simulink model "c221106_FCEV_SLMP_SQP"  (R2022b)
settings: Solver=FixedStepAuto  StartTime=0.0  StopTime=DrvCycLen  FixedStep=1  RelTol=1e-3
values from neighbouring files (symbols this model uses):
  AccThrshd = 1    [Config_c221112.m]    (also in Config_c221127.m; Config_c221218.m; Config_c230117.m; Config_c230321.m)
  AlphaRampFactor = 8    [Config_c221112.m]    (also in Config_c221127.m; Config_c221218.m; Config_c230117.m; Config_c230321.m)
  Bat_eff_chg_average = 0.969    [FCEV_original_data.mat]
  Bat_eff_dis_average = 0.9632    [FCEV_original_data.mat]
  Bat_end_of_life_percent = 20    [FCEV_original_data.mat]
  Bat_I_chg_max = -120    [FCEV_original_data.mat]
  Bat_I_dis_max = 200    [FCEV_original_data.mat]
  Bat_nom_Ic = 2.5    [FCEV_original_data.mat]
  Bat_nom_SOC = 0.35    [FCEV_original_data.mat]
  Bat_nom_temp_oC = 25    [FCEV_original_data.mat]
  Bat_num_pa = 9    [FCEV_original_data.mat]
  Bat_num_se = 97    [FCEV_original_data.mat]
  Bat_ori_C1_chg_F = [397.526659684 455.660832136 435.08783522 460.845064365 457.605812374 417.289828504 416.373906992 359.741413056 321.561704819 1109.14132554 1165.67733205 1135.97600211 ... (72 elements, 9x8)]    [FCEV_original_data.mat]
  Bat_ori_C1_dis_F = [187.121968588 287.083505726 346.448009002 395.529439835 387.517274826 389.973134196 432.856765051 486.92921923 512.158935268 425.990733989 614.68708868 771.472592368 ... (72 elements, 9x8)]    [FCEV_original_data.mat]
  Bat_ori_C2_chg_F = [8748.48589695 7773.35875681 9404.86567646 8934.73981058 8290.58671366 7592.78422269 7759.44623103 7396.59043829 6151.35152293 16187.7227039 11721.8480541 13157.8579836 ... (72 elements, 9x8)]    [FCEV_original_data.mat]
  Bat_ori_C2_dis_F = [2939.81325553 4590.73311898 5504.93546413 5887.5077374 6534.37836712 7765.46899768 10584.7751706 10372.0508438 9238.72693885 5207.86390693 7911.43744944 8879.62137571 ... (72 elements, 9x8)]    [FCEV_original_data.mat]
  Bat_ori_cap_max_Ah = 20.7    [Config_c221218.m]    (also in Config_c230117.m; Config_c230321.m; FCEV_original_data.mat)
  Bat_ori_dUdt4 = [-0.303773584906 -0.249056603774 -0.115094339623 -0.0396226415094 0.0396226415094 0.0641509433962 0.107547169811 0.111320754717 0.0415094339623 0.0547169811321 0.130188679245]    [FCEV_original_data.mat]
  Bat_ori_R0_chg_O = [0.0771669453735 0.0731809311402 0.0726556782939 0.0729965156794 0.0731758310684 0.0742031005051 0.0721266921026 0.0714211058078 0.0714186176143 0.0374124505155 0.0354566732504 0.0345430657188 ... (72 elements, 9x8)]    [FCEV_original_data.mat]
  Bat_ori_R0_dis_O = [0.0819458671157 0.0812429476608 0.0803749674507 0.0805513601722 0.0838629023857 0.0850797840015 0.0829875518672 0.0826388888889 0.0812514106148 0.0428124986417 0.0424658903711 0.0428572670451 ... (72 elements, 9x8)]    [FCEV_original_data.mat]
  Bat_ori_R1_chg_O = [0.114339870884 0.105392753268 0.104421193553 0.109821896183 0.114868279838 0.123333154908 0.129174812826 0.149917249373 0.174896487845 0.0420560161846 0.0390948352938 0.0370122837364 ... (72 elements, 9x8)]    [FCEV_original_data.mat]
  Bat_ori_R1_dis_O = [0.304806399643 0.213604089624 0.171463520004 0.151183840498 0.140630862434 0.128795299077 0.116857791733 0.112567113582 0.106368362501 0.0943235089866 0.0730697254134 0.0611414736086 ... (72 elements, 9x8)]    [FCEV_original_data.mat]
  Bat_ori_R2_chg_O = [0.134518959939 0.17565045702 0.161100627268 0.189032232545 0.205639040497 0.226170473035 0.223651875822 0.181765694192 0.212966950836 0.073628872144 0.0788540822416 0.0792414571734 ... (72 elements, 9x8)]    [FCEV_original_data.mat]
  Bat_ori_R2_dis_O = [0.354968099904 0.285293035102 0.286338708953 0.298763853987 0.248762838155 0.178586175471 0.129047399775 0.188406991173 0.174494800676 0.131839238891 0.123225430215 0.132069033134 ... (72 elements, 9x8)]    [FCEV_original_data.mat]
  Bat_ori_SOC2 = [0 0.001 0.002 0.003 0.004 0.005 0.006 0.007 0.008 0.009 0.01 0.011 ... (1001 elements, 1x1001)]    [FCEV_original_data.mat]
  Bat_ori_SOC4 = [-0.00598301069999 0.0920117618231 0.190864167279 0.289083557951 0.387343788287 0.485011843502 0.5850485992 0.678163031937 0.774810095565 0.876684636119 0.972739524626]    [FCEV_original_data.mat]
  Bat_ori_Uoc_chg_V = [2.4478 2.54923264342 2.6007 2.6383 2.66953057366 2.69636321708 2.7197 2.74042850391 2.75906114733 2.77619379074 2.792 2.80675907757 ... (1001 elements, 1x1001)]    [FCEV_original_data.mat]
  Bat_ori_Uoc_dis_V = [1.9998 2.03916768329 2.24724374236 2.39700902919 2.48767431602 2.5476 2.5882 2.6202 2.64771773167 2.6719 2.6933 2.71251566192 ... (1001 elements, 1x1001)]    [FCEV_original_data.mat]
  Bat_ori_Uoc_V = [2.2238 2.29420016335 2.42397187118 2.5176545146 2.57860244484 2.62198160854 2.65395 2.68031425195 2.7033894395 2.72404689537 2.74265 2.75963736975 ... (1001 elements, 1x1001)]    [FCEV_original_data.mat]
  Bat_power_max_kW = 50    [FCEV_original_data.mat]
  Bat_power_min_kW = 0    [FCEV_original_data.mat]
  Bat_single_capacity_nom_Ah = 2.3    [FCEV_original_data.mat]
  Bat_SOC_ini = 0.3    [Config_c22100601.m]    (also in Config_c22100701.m; FCEV_original_data.mat = 0.45)
  Bat_SOC_max = 0.9    [FCEV_original_data.mat]
  Bat_SOC_min = 0.3    [FCEV_original_data.mat]
  Bat_temp_amb_oC = 25    [FCEV_original_data.mat]
  Bat_temp_cool_oC = 25    [FCEV_original_data.mat]
  BattSocInit = 0.9    [Config_c221112.m]    (also in Config_c221127.m = 0.3; Config_c221218.m = 0.3; Config_c230117.m = 0.8; Config_c230321.m = 0.8)
  BattSocLowerLimit = 0.25    [Config_c221112.m]    (also in Config_c221127.m = 0.3; Config_c221218.m = 0.3; Config_c230117.m = 0.3; Config_c230321.m = 0.3)
  BattSocUpperLimit = 0.9    [Config_c221112.m]    (also in Config_c221127.m = 0.8; Config_c221218.m = 0.8; Config_c230117.m = 0.8; Config_c230321.m = 0.8)
  BattValuePlaceholder = 0    [Config_c221112.m]
  DCAC_eff = 0.95    [FCEV_original_data.mat]
  DCDC_ori_eff = [0.95 0.96 0.97 0.976 0.98 0.978 0.973 0.962]    [FCEV_original_data.mat]
  DCDC_ori_power_kW = [0 10 20 30 40 50 60 70]    [FCEV_original_data.mat]
  DeAccThrshd = -1    [Config_c221112.m]    (also in Config_c221127.m; Config_c221218.m; Config_c230117.m; Config_c230321.m)
  DrvCycRange = sum(DrvCycVps(:,2))    [Config_c221112.m]    (also in Config_c221127.m; Config_c221218.m; Config_c230117.m; Config_c230321.m)
  FC_ori_eff = [0.1 0.33 0.492 0.533 0.559 0.596 0.591 0.562 0.508]    [FCEV_original_data.mat]
  FC_ori_fuel_rate_gps = [0 0.0505050505051 0.0846883468835 0.117260787992 0.149075730471 0.279642058166 0.423011844332 0.593119810202 0.820209973753]    [FCEV_original_data.mat]
  FC_ori_power_kW = [0 2 5 7.5 10 20 30 40 50]    [FCEV_original_data.mat]
  FC_power_max_kW = 50    [FCEV_original_data.mat]
  FC_power_min_kW = 0    [FCEV_original_data.mat]
  m = Time_sample    [Config_c22100601.m]    (also in Config_c22100701.m)
  MC_eff_brk_average = 0.810578512397    [FCEV_original_data.mat]
  MC_eff_dri_average = 0.810578512397    [FCEV_original_data.mat]
  MC_inertia = 0.06    [FCEV_original_data.mat]
  MC_ori_eff = [0.7 0.78 0.85 0.86 0.81 0.82 0.79 0.78 0.78 0.78 0.78 0.7 ... (231 elements, 11x21)]    [FCEV_original_data.mat]
  MC_ori_power_brk_req_kW = [0 -28.3912930389 -56.7825860779 -85.1738791168 -113.565172156 -141.956465195 -170.347758234 -198.739051273 -227.130344311 -255.52163735 -283.912930389 0 ... (121 elements, 11x11)]    [FCEV_original_data.mat]
  MC_ori_power_dri_req_kW = [0 0 0 0 0 0 0 0 0 0 0 0 ... (121 elements, 11x11)]    [FCEV_original_data.mat]
  MC_ori_spd_rpm = [0 1000 2000 3000 4000 5000 6000 7000 8000 9000 10000]    [FCEV_original_data.mat]
  MC_ori_trq_brk_max_Nm = [-271.1368 -271.1368 -271.1368 -237.5159 -178.1369 -142.4824 -118.7579 -101.8119 -89.0685 -79.172 -71.1734]    [FCEV_original_data.mat]
  MC_ori_trq_brk_Nm = [-271.136848522 -244.02316367 -216.909478817 -189.795793965 -162.682109113 -135.568424261 -108.454739409 -81.3410545565 -54.2273697044 -27.1136848522 0]    [FCEV_original_data.mat]
  MC_ori_trq_dri_max_Nm = [271.1368 271.1368 271.1368 237.5159 178.1369 142.4824 118.7579 101.8119 89.0685 79.172 71.1734]    [FCEV_original_data.mat]
  MC_ori_trq_dri_Nm = [0 27.1136848522 54.2273697044 81.3410545565 108.454739409 135.568424261 162.682109113 189.795793965 216.909478817 244.02316367 271.136848522]    [FCEV_original_data.mat]
  MC_ori_trq_Nm = [-271.136848522 -244.02316367 -216.909478817 -189.795793965 -162.682109113 -135.568424261 -108.454739409 -81.3410545565 -54.2273697044 -27.1136848522 0 27.1136848522 ... (21 elements, 1x21)]    [FCEV_original_data.mat]
  MC_power_max_kW = 75    [FCEV_original_data.mat]
  MC_spd_max_rpm = 10000    [FCEV_original_data.mat]
  MC_spd_min_rpm = 0    [FCEV_original_data.mat]
  MC_spd_scale = 1    [FCEV_original_data.mat]
  MC_trq_scale = 1    [FCEV_original_data.mat]
  MC_U_min_V = 120    [FCEV_original_data.mat]
  PredLen = 5    [Config_c221112.m]    (also in Config_c221127.m; Config_c221218.m; Config_c230117.m; Config_c230321.m)
  Road_u = 0.75    [FCEV_original_data.mat]
  SC_np = 1    [Config_c230321.m]
  SC_ns = 100    [Config_c230321.m]
  SC_rc = 1000    [Config_c230321.m]
  SLMP_LearningRate = 0.05    [Config_c221112.m]    (also in Config_c221127.m; Config_c221218.m; Config_c230117.m; Config_c230321.m)
  usd2rmb = 7.116    [Config_c22100601.m]    (also in Config_c22100701.m; Config_c221106.m = 6; Config_c221112.m = 6; Config_c221127.m = 6)
  Veh_air_density_kgpm2 = 1.2    [FCEV_original_data.mat]
  Veh_brk_front = [1 0.6 0.608 0.61 0.618 0.624 0.636 0.645 0.655]    [FCEV_original_data.mat]
  Veh_brk_z = [0.1 0.2 0.3 0.4 0.5 0.6 0.7 0.8 0.9]    [FCEV_original_data.mat]
  Veh_brk_z_max = 0.7    [FCEV_original_data.mat]
  Veh_brk_z_min = 0.1    [FCEV_original_data.mat]
  Veh_coeff_drag = 0.312    [FCEV_original_data.mat]
  Veh_coeff_roll = 0.00863    [FCEV_original_data.mat]
  Veh_final_drive_inertia = 0.1105    [FCEV_original_data.mat]
  Veh_final_drive_ratio = 3.47    [FCEV_original_data.mat]
  Veh_frontal_area_m2 = 2.06    [FCEV_original_data.mat]
  Veh_gravity_acc_ms2 = 9.81    [FCEV_original_data.mat]
  Veh_mass_cargo_kg = 113    [FCEV_original_data.mat]
  Veh_mass_curb_kg = 1157    [FCEV_original_data.mat]
  Veh_mech_eff = 0.9    [FCEV_original_data.mat]
  Veh_rotary_mass_conversion_factor = 1.05    [FCEV_original_data.mat]
  Veh_size_cg_height_m = 0.53    [FCEV_original_data.mat]
  Veh_wheel_inertia = 3.1039    [FCEV_original_data.mat]
  Veh_wheel_radius_m = 0.313    [FCEV_original_data.mat]
  Veh_wt_frac_front = 0.5    [FCEV_original_data.mat]
  VstdThrshd = 2    [Config_c221112.m]    (also in Config_c221127.m; Config_c221218.m; Config_c230117.m; Config_c230321.m)
undefined symbols (not defined in the file or in its folder): Bat_ori_temp, SC_iv, SC_nm, SC_SocTable
libraries: autolibshared x1
(part 1 of 8)
settings Model: Creator=xuupp  LastModifiedBy=xuupp
settings DataIOCC: ReturnWorkspaceOutputs=off
settings RTWCC: GenCodeOnly=on

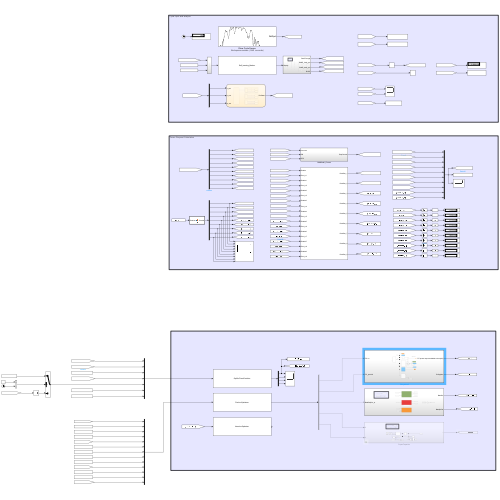
[thumbnail: Simulink's stored preview of the top-level diagram]
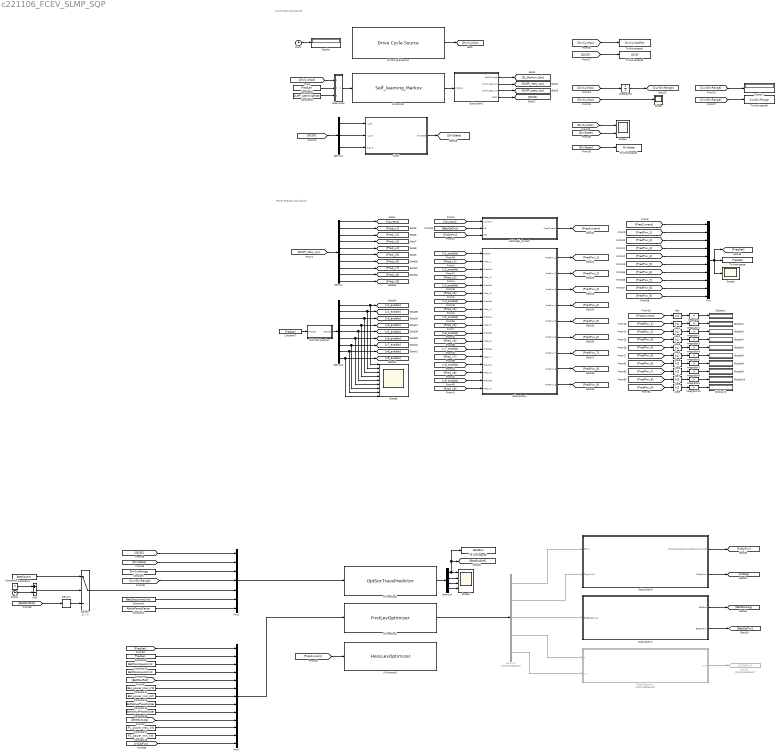
== system c221106_FCEV_SLMP_SQP ==
  note: Power Request Calculation
  note: Cycle input and analyse
  Abs{,1..9} (10 alike) : Abs  SaturateOnIntegerOverflow=off
  Add : Sum  Inputs=+-
  Chart : Stateflow chart  TreatAsAtomicUnit=on
  Clock : Clock
  Clock1 : Clock
  Constant : Constant  Value=DrvCycRange
  Constant1 : Constant  Value=BattSocLowerLimit
  Constant10 : Constant  Value=BattSocUpperLimit
  Constant12 : Constant  Value=Bat_power_max_kW
  Constant13 : Constant  Value=Bat_power_min_kW
  Constant15 : Constant  Value=BattValuePlaceholder
  Constant16 : Constant  Value=BattValuePlaceholder
  Constant17 : Constant  Value=FC_power_max_kW
  Constant18 : Constant  Value=FC_power_min_kW
  Constant2 : Constant  Value=AlphaRampFactor
  Constant3 : Constant  Value=2
  Constant4 : Constant  Value=BattSocInit
  Constant5 : Constant  Value=PredLen
  Constant6 : Constant  Value=SLMP_LearningRate
  Constant7 : Constant  Value=PredLen
  Constant8 : Constant  Value=PredLen
  Constant9 : Constant  Value=BattSocLowerLimit
  Demux : Demux  Outputs=10
  Demux1 : Demux  Outputs=3
  Demux2 : Demux  Commented=on  Outputs=5
  Demux3 : Demux
  Demux4 : Demux  Outputs=9
  Display{,1..11} (12 alike) : Display
  Drive Cycle Source : autolibshared/Drive Cycle Source  cycleVar=Workspace variable  wsVar=DrvCycVps  fileVar=cycleFTP75.mat  tfinal="1640  seconds"  cycleRepeat=off  outAccPort=off  outGearPort=off  gearList=No gear data  t_wot1=5  xdot_woto=0  xdot_wot1=30  t_wot2=20  xdot_wot2=0  t_wotend=30  srcUnit=m/s  outUnit=m/s  srcAccUnit=m/s/s  outAccUnit=m/s^2  dt=1  aMode=1  faultOption=off  velBnd=2  velBndUnit=mph  inUnit=m/s  timeBnd=1  failOption=off  stopSim=off  maxFaultCnt=10  maxFaultTime=2  maxTotFaultTime=15  traceOption=off  dtTrace=1  traceWindow=10  lastDCname=Custom Data Set  lastOutUnit=mph  lastDT=1  lastTB=1  lastSB=2  forceCalcBound=off
  Goto21 : Goto  Commented=on  GotoTag=ScOpPwr
  Integrator{,1..10} (11 alike) : Integrator
  MATLAB Function : MATLAB Function  TreatAsAtomicUnit=on
  Memory : Memory  InheritSampleTime=on
  Mux : Mux  Inputs=10
  Mux1 : Mux  Inputs=7
  Mux2 : Mux  Inputs=13
  S-Function : S-Function  FunctionName=Self_learning_Markov  SFunctionDeploymentMode=off  EnableBusSupport=off
  S-Function1 : S-Function  FunctionName=FirstLevOptimizer  SFunctionDeploymentMode=off  EnableBusSupport=off
  S-Function2 : S-Function  FunctionName=OptSocTracePredictor  SFunctionDeploymentMode=off  EnableBusSupport=off
  S-Function3 : S-Function  FunctionName=HessLevOptimizer  SFunctionDeploymentMode=off  EnableBusSupport=off
  Scope : Scope
  Scope1 : Scope
  Scope2 : Scope  NumInputPorts=4
  Scope3 : Scope  NumInputPorts=9
  Scope4 : Scope  NumInputPorts=2
  Subsystem : Subsystem
  Subsystem1 : Subsystem
  Subsystem2 : Subsystem
  Subsystem3 : Subsystem
  Subsystem4 : Subsystem
  SuperCapacitor : Subsystem  Commented=on
  Switch : Switch  Criteria=u2 > Threshold  SaturateOnIntegerOverflow=off  InputSameDT=off
  To Workspace : ToWorkspace  VariableName=PreqSet  SampleTime=-1
  To Workspace1 : ToWorkspace  VariableName=DrvCycVpsRec  SampleTime=-1
  To Workspace2 : ToWorkspace  VariableName=BattSoc  SampleTime=-1
  To Workspace3 : ToWorkspace  VariableName=DCSF  SampleTime=-1
  To Workspace4 : ToWorkspace  VariableName=DrvState  SampleTime=-1
  To Workspace5 : ToWorkspace  VariableName=CurrDrvRange  SampleTime=-1
  VehModel_Current : Subsystem
  wires:
  S-Function/1 -> Subsystem1/1(Display)
  [DrvCycVps] -> Subsystem/1(RowSequence)
  Drive Cycle Source/1 -> [DrvCycVps]
  Clock/1 -> Display/1
  Subsystem1/3(SLMP_aset_vps) -> [SLMP_aset_vps]
  Subsystem/1(HstLog) -> S-Function/1
  Subsystem1/1(PassThrough) -> [SL_Markov_Set]
  Subsystem1/2(SLMP_Vset_vps) -> [SLMP_Vset_vps]
  [SLMP_Vset_vps] -> Demux/1
  Demux/1 -> [Vcurrent]
  Demux/2 -> [Pred_v1]
  Demux/3 -> [Pred_v2]
  Demux/4 -> [Pred_v3]
  Demux/5 -> [Pred_v4]
  Demux/6 -> [Pred_v5]
  [Vcurrent] -> VehModel_Current/1(Vcurrent)
  VehModel_Current/1(PreqCurrent) -> [PreqCurrent]
  [PreqCurrent] -> Mux/1
  [PredPwr_1] -> Mux/2
  [PredPwr_2] -> Mux/3
  [PredPwr_3] -> Mux/4
  [PredPwr_4] -> Mux/5
  [PredPwr_5] -> Mux/6
  Mux/1 -> Scope1/1, [PreqSet], To Workspace/1
  [PreqCurrent] -> Abs/1
  [PredPwr_1] -> Abs1/1
  [PredPwr_2] -> Abs2/1
  [PredPwr_3] -> Abs3/1
  [PredPwr_4] -> Abs4/1
  [PredPwr_5] -> Abs5/1
  Abs/1 -> Integrator/1
  Integrator/1 -> Display1/1
  Abs1/1 -> Integrator1/1
  Abs2/1 -> Integrator2/1
  Abs3/1 -> Integrator3/1
  Abs4/1 -> Integrator4/1
  Abs5/1 -> Integrator5/1
  Integrator1/1 -> Display2/1
  Integrator2/1 -> Display3/1
  Integrator3/1 -> Display4/1
  Integrator4/1 -> Display5/1
  Integrator5/1 -> Display6/1
  [BattOpPwr] -> VehModel_Current/2(PB)
  [FcOpPwr] -> VehModel_Current/3(PFC)
  [DCSF] -> Demux1/1
  [DrvCycVps] -> Scope/1
  [DrvCycVps] -> Integrator6/1
  [DrvCycVps] -> To Workspace1/1
  Subsystem1/4(DCSF) -> [DCSF]
  [DCSF] -> To Workspace3/1
  Demux1/1 -> Chart/1(v_std)
  Demux1/2 -> Chart/2(v_ave)
  Demux1/3 -> Chart/3(a_ave)
  Chart/1(DrvState) -> [DrvState]
  [DrvCycVps] -> Scope4/1
  [DrvState] -> Scope4/2
  [DrvState] -> To Workspace4/1
  S-Function1/1 -> Demux2/1
  Demux2/1 -> Subsystem3/1(FC on)
  Demux2/2 -> Subsystem3/2("FC_pwr kW ")
  Demux2/4 -> SuperCapacitor/1(P)
  Demux2/5 -> SuperCapacitor/2(In2)
  Subsystem3/1(FC power output avaliable to bus (kW)) -> [FcOpPwr]
  SuperCapacitor/1(Out1) -> Goto21/1
  Subsystem3/2(FcDegMux) -> [FcDeg]
  Mux2/1 -> S-Function1/1
  [PreqCurrent] -> S-Function3/1
  Integrator6/1 -> [CurrDrvRange]
  [CurrDrvRange] -> Display7/1
  Demux2/3 -> Subsystem2/1(BattReqPwr_w)
  Subsystem2/2(BattOpPwr) -> [BattOpPwr]
  Subsystem2/1(BattSoc) -> [BattSocLog]
  Mux1/1 -> S-Function2/1
  S-Function2/1 -> Demux3/1
  Demux3/1 -> [BattSocRef], To Workspace2/1, Scope2/1
  Demux3/2 -> Scope2/2
  Demux3/3 -> Scope2/3
  Constant2/1 -> Mux1/7
  Clock1/1 -> Add/2
  Constant3/1 -> Add/1
  [BattSocRef] -> Memory/1
  Add/1 -> Switch/2
  Constant1/1 -> Mux1/6
  Constant/1 -> Mux1/3
  [DCSF] -> Mux1/1
  [CurrDrvRange] -> Mux1/4
  Constant4/1 -> Switch/1
  [DrvState] -> Mux1/2
  Switch/1 -> Mux1/5
  Demux3/4 -> Scope2/4
  Memory/1 -> Switch/3
  [CurrDrvRange] -> To Workspace5/1
  Constant5/1 -> Subsystem/2(RowSequence1)
  Constant6/1 -> Subsystem/3(RowSequence2)
  Demux/7 -> [Pred_v6]
  Demux/8 -> [Pred_v7]
  Demux/9 -> [Pred_v8]
  Demux/10 -> [Pred_v9]
  Constant7/1 -> MATLAB Function/1(PredLen)
  MATLAB Function/1(Enable) -> Demux4/1
  Demux4/1 -> Scope3/1, [v1_enable]
  Demux4/2 -> Scope3/2, [v2_enable]
  Demux4/3 -> Scope3/3, [v3_enable]
  Demux4/4 -> Scope3/4, [v4_enable]
  Demux4/5 -> Scope3/5, [v5_enable]
  Demux4/6 -> Scope3/6, [v6_enable]
  Demux4/7 -> Scope3/7, [v7_enable]
  Demux4/8 -> Scope3/8, [v8_enable]
  Demux4/9 -> Scope3/9, [v9_enable]
  [v1_enable] -> Subsystem4/1(Enable)
  [Pred_v1] -> Subsystem4/2(Pred_v1)
  [v2_enable] -> Subsystem4/3(Enable1)
  [Pred_v2] -> Subsystem4/4(Pred_v2)
  [v3_enable] -> Subsystem4/5(Enable2)
  [Pred_v3] -> Subsystem4/6(Pred_v3)
  [v4_enable] -> Subsystem4/7(Enable3)
  [Pred_v4] -> Subsystem4/8(Pred_v4)
  [v5_enable] -> Subsystem4/9(Enable4)
  [Pred_v5] -> Subsystem4/10(Pred_v5)
  [v6_enable] -> Subsystem4/11(Enable5)
  [Pred_v6] -> Subsystem4/12(Pred_v6)
  [v7_enable] -> Subsystem4/13(Enable6)
  [Pred_v7] -> Subsystem4/14(Pred_v7)
  [v8_enable] -> Subsystem4/15(Enable7)
  [Pred_v8] -> Subsystem4/16(Pred_v8)
  [v9_enable] -> Subsystem4/17(Enable8)
  [Pred_v9] -> Subsystem4/18(Pred_v9)
  Subsystem4/1(PredPwr_1) -> [PredPwr_1]
  Subsystem4/2(PredPwr_2) -> [PredPwr_2]
  Subsystem4/3(PredPwr_3) -> [PredPwr_3]
  Subsystem4/4(PredPwr_4) -> [PredPwr_4]
  Subsystem4/5(PredPwr_5) -> [PredPwr_5]
  Subsystem4/6(PredPwr_6) -> [PredPwr_6]
  Subsystem4/7(PredPwr_7) -> [PredPwr_7]
  Subsystem4/8(PredPwr_8) -> [PredPwr_8]
  Subsystem4/9(PredPwr_9) -> [PredPwr_9]
  [PredPwr_6] -> Abs6/1
  Abs6/1 -> Integrator7/1
  Integrator7/1 -> Display8/1
  Integrator8/1 -> Display9/1
  Abs7/1 -> Integrator8/1
  Abs8/1 -> Integrator9/1
  Integrator9/1 -> Display10/1
  Integrator10/1 -> Display11/1
  Abs9/1 -> Integrator10/1
  [PredPwr_7] -> Abs7/1
  [PredPwr_8] -> Abs8/1
  [PredPwr_9] -> Abs9/1
  [PredPwr_6] -> Mux/7
  [PredPwr_7] -> Mux/8
  [PredPwr_8] -> Mux/9
  [PredPwr_9] -> Mux/10
  [PreqSet] -> Mux2/1
  Constant8/1 -> Mux2/2
  Constant10/1 -> Mux2/3
  Constant9/1 -> Mux2/4
  [BattSocRef] -> Mux2/5
  Constant12/1 -> Mux2/6
  Constant13/1 -> Mux2/7
  Constant15/1 -> Mux2/8
  Constant16/1 -> Mux2/9
  [BattSocLog] -> Mux2/10
  Constant17/1 -> Mux2/11
  Constant18/1 -> Mux2/12
  [FcOpPwr] -> Mux2/13

== system c221106_FCEV_SLMP_SQP/Subsystem ==
  RowSequence : Inport
  RowSequence1 : Inport  Port=2
  RowSequence2 : Inport  Port=3
  Delay : Delay  DelayLength=1
  Delay1 : Delay
  Delay2 : Delay  DelayLength=3
  Delay3 : Delay  DelayLength=4
  Delay4 : Delay  DelayLength=5
  Delay5 : Delay  DelayLength=6
  Delay6 : Delay  DelayLength=7
  Delay7 : Delay  DelayLength=8
  Delay8 : Delay  DelayLength=9
  Mux : Mux  Inputs=12
  HstLog : Outport
  wires:
  RowSequence/1 -> Delay8/1, Delay7/1, Delay6/1, Delay5/1, Delay4/1, Delay3/1, Delay2/1, Delay1/1, Delay/1, Mux/1
  Mux/1 -> HstLog/1
  Delay8/1 -> Mux/10
  Delay7/1 -> Mux/9
  Delay6/1 -> Mux/8
  Delay5/1 -> Mux/7
  Delay3/1 -> Mux/5
  Delay2/1 -> Mux/4
  Delay1/1 -> Mux/3
  Delay/1 -> Mux/2
  Delay4/1 -> Mux/6
  RowSequence1/1 -> Mux/11
  RowSequence2/1 -> Mux/12

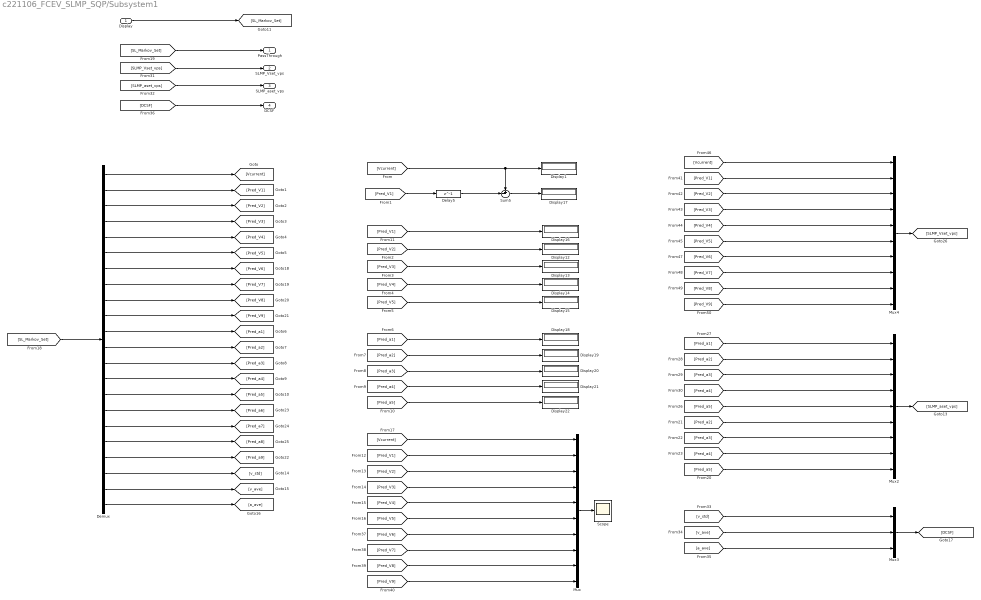
== system c221106_FCEV_SLMP_SQP/Subsystem1 ==
  Display : Inport
  Delay5 : Delay  DelayLength=1
  Demux : Demux  Outputs=22
  Display{1,12..22} (12 alike) : Display
  Mux : Mux  Inputs=10
  Mux2 : Mux  Inputs=9
  Mux3 : Mux  Inputs=3
  Mux4 : Mux  Inputs=10
  Scope : Scope
  Sum5 : Sum  Inputs=+-|
  PassThrough : Outport
  SLMP_Vset_vps : Outport  Port=2
  SLMP_aset_vps : Outport  Port=3
  DCSF : Outport  Port=4
  wires:
  Display/1 -> [SL_Markov_Set]
  Demux/1 -> [Vcurrent]
  Demux/2 -> [Pred_V1]
  Demux/3 -> [Pred_V2]
  Demux/4 -> [Pred_V3]
  Demux/5 -> [Pred_V4]
  Demux/6 -> [Pred_V5]
  [Pred_V1] -> Delay5/1
  Delay5/1 -> Sum5/2
  [Pred_V2] -> Display12/1
  [Pred_V3] -> Display13/1
  [Vcurrent] -> Display1/1, Sum5/1
  Sum5/1 -> Display17/1
  [Pred_V4] -> Display14/1
  [Pred_V5] -> Display15/1
  [Pred_V1] -> Display16/1
  [Pred_a1] -> Display18/1
  [Pred_a2] -> Display19/1
  [Pred_a3] -> Display20/1
  [Pred_a4] -> Display21/1
  [Pred_a5] -> Display22/1
  Mux/1 -> Scope/1
  [Pred_V5] -> Mux/6
  [Pred_V4] -> Mux/5
  [Pred_V3] -> Mux/4
  [Pred_V2] -> Mux/3
  [Pred_V1] -> Mux/2
  [Vcurrent] -> Mux/1
  [SL_Markov_Set] -> Demux/1
  [SL_Markov_Set] -> PassThrough/1
  [Pred_a3] -> Mux2/3
  [Pred_a2] -> Mux2/2
  [Pred_a1] -> Mux2/1
  [Pred_a4] -> Mux2/4
  [Pred_a5] -> Mux2/5
  Mux2/1 -> [SLMP_aset_vps]
  [SLMP_Vset_vps] -> SLMP_Vset_vps/1
  [SLMP_aset_vps] -> SLMP_aset_vps/1
  [v_std] -> Mux3/1
  [v_ave] -> Mux3/2
  [a_ave] -> Mux3/3
  Mux3/1 -> [DCSF]
  [DCSF] -> DCSF/1
  Demux/7 -> [Pred_V6]
  Demux/8 -> [Pred_V7]
  Demux/9 -> [Pred_V8]
  Demux/10 -> [Pred_V9]
  Demux/11 -> [Pred_a1]
  Demux/12 -> [Pred_a2]
  Demux/13 -> [Pred_a3]
  Demux/14 -> [Pred_a4]
  Demux/15 -> [Pred_a5]
  Demux/16 -> [Pred_a6]
  Demux/17 -> [Pred_a7]
  Demux/18 -> [Pred_a8]
  Demux/19 -> [Pred_a9]
  Demux/20 -> [v_std]
  Demux/21 -> [v_ave]
  Demux/22 -> [a_ave]
  [Pred_V6] -> Mux/7
  [Pred_V9] -> Mux/10
  [Pred_V7] -> Mux/8
  [Pred_V8] -> Mux/9
  [Pred_V8] -> Mux4/9
  [Pred_V7] -> Mux4/8
  [Pred_V9] -> Mux4/10
  [Pred_V6] -> Mux4/7
  [Vcurrent] -> Mux4/1
  [Pred_V1] -> Mux4/2
  [Pred_V2] -> Mux4/3
  [Pred_V3] -> Mux4/4
  [Pred_V4] -> Mux4/5
  [Pred_V5] -> Mux4/6
  Mux4/1 -> [SLMP_Vset_vps]
  [Pred_a2] -> Mux2/6
  [Pred_a3] -> Mux2/7
  [Pred_a4] -> Mux2/8
  [Pred_a5] -> Mux2/9

== system c221106_FCEV_SLMP_SQP/Subsystem2 ==
  note: Thermal Model (Cell)
  note: Electrical Model
  BattReqPwr_w : Inport
  Add : Sum
  Capacity Degradation Model (Cell)1 : Subsystem
  Electrical Model1 : Subsystem  Tag=electrical
  Gain : Gain  Gain=0.5
  Thermal Model1 : Subsystem
  BattSoc : Outport
  BattOpPwr : Outport  Port=2
  wires:
  [BattReqPwr_w] -> Electrical Model1/2(Pb,r)
  Electrical Model1/4(Pb,ava) -> [BattOpPwr]
  Thermal Model1/2(Ts.) -> [BattTemp_s]
  Electrical Model1/2(SOC) -> [BattSoc]
  Electrical Model1/3(I) -> [BattCurrent]
  [BattTemp] -> Electrical Model1/1(T)
  [BattTemp] -> Capacity Degradation Model (Cell)1/1(Temp (oC))
  [BattCurrent] -> Capacity Degradation Model (Cell)1/3(I(A))
  [BattSoc] -> Capacity Degradation Model (Cell)1/2(SOC)
  Electrical Model1/1(Qb) -> [Batt_Qb]
  [Batt_Qb] -> Thermal Model1/1(Qb)
  Thermal Model1/1(Tc.) -> [BattTemp_c]
  [BattTemp_c] -> Add/2
  [BattTemp_s] -> Add/1
  Add/1 -> Gain/1
  Gain/1 -> [BattTemp]
  BattReqPwr_w/1 -> [BattReqPwr_w]
  [BattSoc] -> BattSoc/1
  [BattOpPwr] -> BattOpPwr/1

== system c221106_FCEV_SLMP_SQP/Subsystem3 ==
  note: Direct Hydrogen PEM Fuel Cell
  note: Note: Speed NOT used; carried only for compatability.
  note: 不虑DC/DC转换器
  FC on : Inport
  "FC_pwr kW " : Inport  Port=2
  Add : Sum
  DC/DC efficiency : Lookup_n-D  NumberOfTableDimensions=1  BreakpointsForDimension1=DCDC_ori_power_kW  Table=DCDC_ori_eff  RndMeth=Simplest
  Display7 : Display
  Divide2 : Product  Inputs=**
  FcDegCountingSubSys : Subsystem
  Fuel Rate Calculation1 : Subsystem
  Fuel cell efficiency calculation : Subsystem
  Gain : Gain  Gain=1/1000
  Memory : Memory  InheritSampleTime=on
  Power Calculation : Subsystem
  Saturation1 : Saturate  UpperLimit=FC_power_max_kW  LowerLimit=FC_power_min_kW
  Saturation2 : Saturate  UpperLimit=FC_power_max_kW  LowerLimit=FC_power_min_kW
  Scope{,2..3,6} (4 alike) : Scope
  To Workspace1 : ToWorkspace  VariableName=FC_fuel_consume_kg  SampleTime=-1
  To Workspace5 : ToWorkspace  VariableName=FC_eff  SampleTime=-1
  To Workspace9 : ToWorkspace  VariableName=FC_power_kW  SampleTime=-1
  FC power output avaliable to bus (kW) : Outport
  FcDegMux : Outport  Port=2
  tag scope: FC_fuel_consume_kg=global, FC_fuel_rate_gps=global, FC_power_kW=global
  wires:
  Saturation2/1 -> FcDegCountingSubSys/1(P_fc), Fuel cell efficiency calculation/1(fc power)
  Divide2/1 -> FC power output avaliable to bus (kW)/1
  Fuel Rate Calculation1/1(fcv_H2_rate (g/s)1) -> [FC_fuel_rate_gps], Scope3/1, Add/1
  Add/1 -> Memory/1, Gain/1
  Fuel cell efficiency calculation/1("fc_eff ") -> To Workspace5/1
  Saturation1/1 -> DC/DC efficiency/1, Scope2/1, [FC_power_kW], To Workspace9/1, Divide2/2, Saturation2/1, Fuel Rate Calculation1/1(fc pwr)
  FcDegCountingSubSys/2(FcDegSum) -> Display7/1, Scope/1
  Memory/1 -> Add/2
  FcDegCountingSubSys/1(FcDegMux) -> FcDegMux/1
  DC/DC efficiency/1 -> Divide2/1
  Gain/1 -> Scope6/1, To Workspace1/1, [FC_fuel_consume_kg]
  FC on/1 -> Power Calculation/1(fc on)
  Power Calculation/1(Power output (kW)) -> Saturation1/1
  "FC_pwr kW "/1 -> Power Calculation/2(Power command (kW))

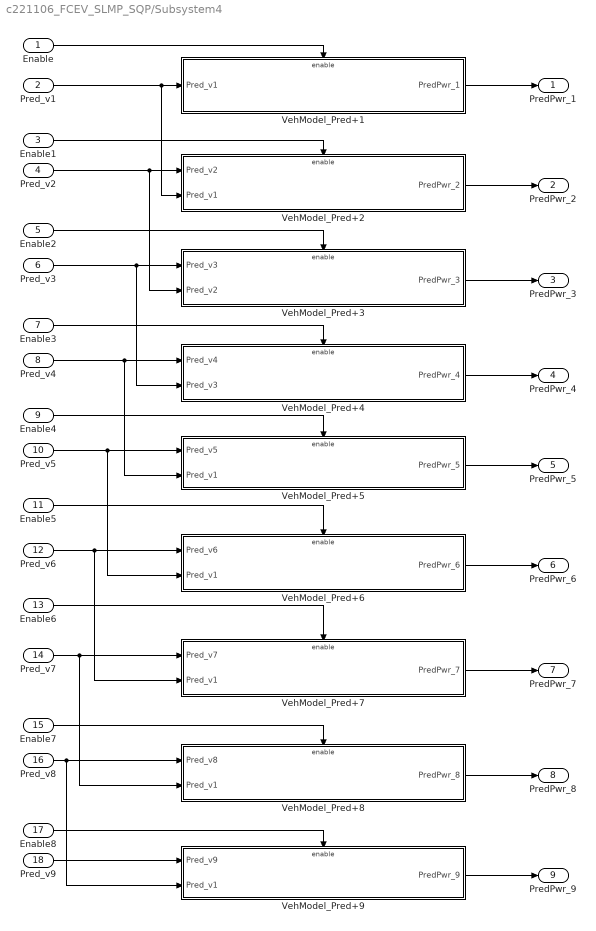
== system c221106_FCEV_SLMP_SQP/Subsystem4 ==
  Enable : Inport
  Pred_v1 : Inport  Port=2
  Enable1 : Inport  Port=3
  Pred_v2 : Inport  Port=4
  Enable2 : Inport  Port=5
  Pred_v3 : Inport  Port=6
  Enable3 : Inport  Port=7
  Pred_v4 : Inport  Port=8
  Enable4 : Inport  Port=9
  Pred_v5 : Inport  Port=10
  Enable5 : Inport  Port=11
  Pred_v6 : Inport  Port=12
  Enable6 : Inport  Port=13
  Pred_v7 : Inport  Port=14
  Enable7 : Inport  Port=15
  Pred_v8 : Inport  Port=16
  Enable8 : Inport  Port=17
  Pred_v9 : Inport  Port=18
  VehModel_Pred+1 : Subsystem
  VehModel_Pred+2 : Subsystem
  VehModel_Pred+3 : Subsystem
  VehModel_Pred+4 : Subsystem
  VehModel_Pred+5 : Subsystem
  VehModel_Pred+6 : Subsystem
  VehModel_Pred+7 : Subsystem
  VehModel_Pred+8 : Subsystem
  VehModel_Pred+9 : Subsystem
  PredPwr_1 : Outport
  PredPwr_2 : Outport  Port=2
  PredPwr_3 : Outport  Port=3
  PredPwr_4 : Outport  Port=4
  PredPwr_5 : Outport  Port=5
  PredPwr_6 : Outport  Port=6
  PredPwr_7 : Outport  Port=7
  PredPwr_8 : Outport  Port=8
  PredPwr_9 : Outport  Port=9
  wires:
  Pred_v1/1 -> VehModel_Pred+2/2(Pred_v1), VehModel_Pred+1/1(Pred_v1)
  Pred_v3/1 -> VehModel_Pred+4/2(Pred_v3), VehModel_Pred+3/1(Pred_v3)
  Enable7/1 -> VehModel_Pred+8/Enable
  Enable6/1 -> VehModel_Pred+7/Enable
  VehModel_Pred+1/1(PredPwr_1) -> PredPwr_1/1
  Enable8/1 -> VehModel_Pred+9/Enable
  VehModel_Pred+7/1(PredPwr_7) -> PredPwr_7/1
  Enable1/1 -> VehModel_Pred+2/Enable
  VehModel_Pred+6/1(PredPwr_6) -> PredPwr_6/1
  Enable5/1 -> VehModel_Pred+6/Enable
  VehModel_Pred+9/1(PredPwr_9) -> PredPwr_9/1
  VehModel_Pred+3/1(PredPwr_3) -> PredPwr_3/1
  Pred_v9/1 -> VehModel_Pred+9/1(Pred_v9)
  Enable/1 -> VehModel_Pred+1/Enable
  Pred_v5/1 -> VehModel_Pred+6/2(Pred_v1), VehModel_Pred+5/1(Pred_v5)
  Pred_v2/1 -> VehModel_Pred+3/2(Pred_v2), VehModel_Pred+2/1(Pred_v2)
  VehModel_Pred+5/1(PredPwr_5) -> PredPwr_5/1
  VehModel_Pred+4/1(PredPwr_4) -> PredPwr_4/1
  Pred_v7/1 -> VehModel_Pred+7/1(Pred_v7), VehModel_Pred+8/2(Pred_v1)
  Enable3/1 -> VehModel_Pred+4/Enable
  VehModel_Pred+2/1(PredPwr_2) -> PredPwr_2/1
  Pred_v4/1 -> VehModel_Pred+5/2(Pred_v1), VehModel_Pred+4/1(Pred_v4)
  Pred_v8/1 -> VehModel_Pred+8/1(Pred_v8), VehModel_Pred+9/2(Pred_v1)
  VehModel_Pred+8/1(PredPwr_8) -> PredPwr_8/1
  Pred_v6/1 -> VehModel_Pred+7/2(Pred_v1), VehModel_Pred+6/1(Pred_v6)
  Enable4/1 -> VehModel_Pred+5/Enable
  Enable2/1 -> VehModel_Pred+3/Enable

== system c221106_FCEV_SLMP_SQP/SuperCapacitor ==
  P : Inport
  In2 : Inport  Port=2
  Add1 : Sum  Inputs=+-
  Clock1 : Clock
  Constant10 : Constant  Value=20
  Constant11 : Constant  Value=0
  Constant12 : Constant
  Constant13 : Constant  Value=2.4
  Constant14 : Constant  Value=SC_iv
  Constant15 : Constant  Value=SC_rc
  Constant2 : Constant  Value=SC_nm*SC_np*SC_ns
  Constant3 : Constant  Value=6000
  Display2 : Display
  MATLAB Function1 : MATLAB Function  TreatAsAtomicUnit=on
  Manual Switch2 : ManualSwitch  CurrentSetting=0
  Manual Switch3 : ManualSwitch
  Memory1 : Memory
  SC_Volt_2_Soc1 : Lookup_n-D  NumberOfTableDimensions=1  BreakpointsForDimension1=SC_SocTable(:,1)  Table=SC_SocTable(:,2)  InternalRulePriority=Speed  RndMeth=Simplest
  Scope1 : Scope  NumInputPorts=3
  Stop Simulation1 : Stop
  Switch2 : Switch  Criteria=u2 > Threshold  Threshold=1  SaturateOnIntegerOverflow=off  InputSameDT=off
  Switch3 : Switch  Criteria=u2 > Threshold  SaturateOnIntegerOverflow=off  InputSameDT=off
  Out1 : Outport
  wires:
  Switch3/1 -> Stop Simulation1/1
  Constant12/1 -> Switch3/3
  Constant10/1 -> Add1/2
  SC_Volt_2_Soc1/1 -> [SC_soc], Scope1/1, Add1/1
  Constant3/1 -> Manual Switch3/2
  P/1 -> [PwrInput]
  Clock1/1 -> Switch2/2, Display2/1
  MATLAB Function1/1(y) -> SC_Volt_2_Soc1/1, Scope1/2, Memory1/1
  Add1/1 -> Switch3/2
  Constant15/1 -> Manual Switch3/1
  Constant14/1 -> Manual Switch2/1
  Constant11/1 -> Switch3/1
  Constant2/1 -> MATLAB Function1/2(n)
  Manual Switch2/1 -> Switch2/3
  Constant13/1 -> Manual Switch2/2
  Memory1/1 -> Switch2/1
  Switch2/1 -> MATLAB Function1/4(u_k)
  Manual Switch3/1 -> MATLAB Function1/3(c)
  In2/1 -> Scope1/3
  [PwrInput] -> MATLAB Function1/1(P)
  [SC_soc] -> Out1/1

== system c221106_FCEV_SLMP_SQP/VehModel_Current ==
  note: CarryOver
  Vcurrent : Inport
  PB : Inport  Port=2
  PFC : Inport  Port=3
  Gain : Gain  Gain=3.6
  Power bus : Subsystem
  主减及变速器模型 : Subsystem
  整车动力学模型 : Subsystem
  车轮模型 : Subsystem
  驱动电机模型 : Subsystem
  PreqCurrent : Outport
  wires:
  主减及变速器模型/1(drive torque (Nm) speed (rad/s) brike torque (Nm) req'd at input side of final drive) -> 驱动电机模型/1(drive torque (Nm) speed (rad/s) brake torque (Nm) req'd at motor)
  驱动电机模型/1(drive power (kW) brake power (kW) req'd motor input power (电功率)) -> Power bus/1(drive power (kW) brake power (kW) req at power bus)
  驱动电机模型/2(drive torque (Nm) brake torque (Nm) speed avail (rad/s) avail. at rotor) -> 主减及变速器模型/2(drive torque (Nm) brake torque (Nm) speed avail (rad/s) at input side of final drive)
  主减及变速器模型/2(drive torque (Nm) brake torque (Nm) speed avail (rad/s) at output side of final drive) -> 车轮模型/2("drive torque (Nm) brake torque (Nm) speed (rad/s) available from drivetrain into axle ")
  车轮模型/2(tractive force (N) brake force (N) linear speed achievable (m/s)) -> 整车动力学模型/2(实际车辆驱动力N 制动力N 和车速m/s)
  整车动力学模型/1(需求驱动力N 目标车速m/s 需求制动力N) -> 车轮模型/1("tractive force, brake force and speed req'd of tire/road interface 需求驱动力N 目标车速m/s 需求制动力N")
  车轮模型/1(drive torque (Nm) speed (rad/s) brake torque (Nm) req'd from drivetrain into axle) -> 主减及变速器模型/1(drive torque (Nm) speed (rad/s) brake torque (Nm) req'd at output side of final drive)
  Vcurrent/1 -> Gain/1
  Power bus/2(drive power (kW) brake power (kW) availableat power bus) -> 驱动电机模型/2(drive power (kW) brake power (kW) input available motor)
  PB/1 -> Power bus/2(pwr availible from battery kW)
  PFC/1 -> Power bus/3(pwr availible from FC_+DCDC kW)
  Power bus/1(drive power (kW)/brake power (kW) req from power sources) -> PreqCurrent/1
  Gain/1 -> 整车动力学模型/1(需求车速 km/h)

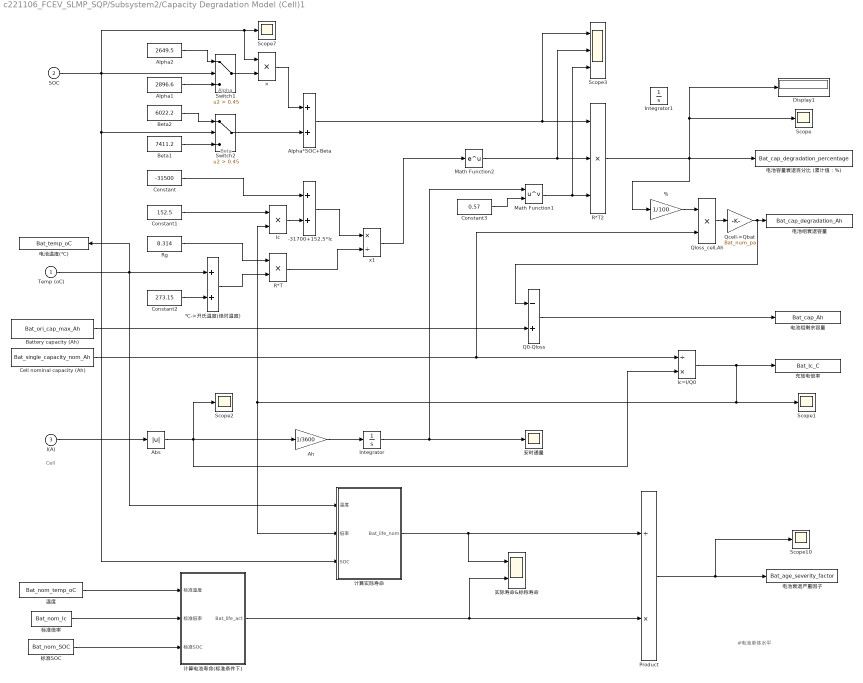
== system c221106_FCEV_SLMP_SQP/Subsystem2/Capacity Degradation Model (Cell)1 ==
  note: Cell
  note: #电池单体水平
  note: Beta
  note: Alpha
  Temp (oC) : Inport
  SOC : Inport  Port=2
  I(A) : Inport  Port=3
  % : Gain  Gain=1/100
  -31700+152.5*Ic : Sum  InputSameDT=on  SaturateOnIntegerOverflow=on  OutDataTypeStr=Inherit: Same as first input
  Abs : Abs  SaturateOnIntegerOverflow=off
  Ah : Gain  Gain=1/3600
  Alpha*SOC+Beta : Sum  InputSameDT=on  SaturateOnIntegerOverflow=on  OutDataTypeStr=Inherit: Same as first input
  Alpha1 : Constant  Value=2896.6
  Alpha2 : Constant  Value=2649.5
  Battery capacity (Ah) : Constant  Value=Bat_ori_cap_max_Ah
  Beta1 : Constant  Value=7411.2
  Beta2 : Constant  Value=6022.2
  Cell nominal capacity (Ah) : Constant  Value=Bat_single_capacity_nom_Ah
  Constant : Constant  Value=-31500
  Constant1 : Constant  Value=152.5
  Constant2 : Constant  Value=273.15
  Constant3 : Constant  Value=0.57
  Display1 : Display
  Ic : Product  InputSameDT=on  RndMeth=Zero  SaturateOnIntegerOverflow=on  OutDataTypeStr=Inherit: Same as first input
  Ic=I/Q0 : Product  Inputs=/*  InputSameDT=on  RndMeth=Zero  SaturateOnIntegerOverflow=on  OutDataTypeStr=Inherit: Same as first input
  Integrator : Integrator  InitialCondition=eps
  Integrator1 : Integrator
  Math Function1 : Math  Operator=pow  SignedPower=on
  Math Function2 : Math  SignedPower=on
  Product : Product  Inputs=/*
  Q0-Qloss : Sum  Inputs=-+  InputSameDT=on  SaturateOnIntegerOverflow=on  OutDataTypeStr=Inherit: Same as first input
  Qcell->Qbat : Gain  Gain=Bat_num_pa  SaturateOnIntegerOverflow=on  OutDataTypeStr=Inherit: Same as input  ParamDataTypeStr=Inherit: Same as input
  Qloss_cell,Ah : Product  InputSameDT=on  RndMeth=Zero  SaturateOnIntegerOverflow=on  OutDataTypeStr=Inherit: Same as first input
  R*T : Product  InputSameDT=on  RndMeth=Zero  SaturateOnIntegerOverflow=on  OutDataTypeStr=Inherit: Same as first input
  R*T2 : Product  Inputs=3  InputSameDT=on  RndMeth=Zero  SaturateOnIntegerOverflow=on  OutDataTypeStr=Inherit: Same as first input
  Rg : Constant  Value=8.314
  Scope{,1..2,7,10} (5 alike) : Scope
  Scope3 : Scope  NumInputPorts=3
  Switch1 : Switch  Criteria=u2 > Threshold  Threshold=0.45
  Switch2 : Switch  Criteria=u2 > Threshold  Threshold=0.45
  x1 : Product  Inputs=*/  InputSameDT=on  RndMeth=Zero  SaturateOnIntegerOverflow=on  OutDataTypeStr=Inherit: Same as first input
  × : Product  InputSameDT=on  RndMeth=Zero  SaturateOnIntegerOverflow=on  OutDataTypeStr=Inherit: Same as first input
  ℃->开氏温度(绝对温度) : Sum  InputSameDT=on  SaturateOnIntegerOverflow=on  OutDataTypeStr=Inherit: Same as first input
  充放电倍率 : ToWorkspace  VariableName=Bat_Ic_C  SampleTime=-1
  安时通量 : Scope
  实际寿命&标称寿命 : Scope  NumInputPorts=2
  标准SOC : Constant  Value=Bat_nom_SOC
  标准倍率 : Constant  Value=Bat_nom_Ic
  温度 : Constant  Value=Bat_nom_temp_oC  VectorParams1D=off
  电池容量衰退百分比 (累计值：%) : ToWorkspace  VariableName=Bat_cap_degradation_percentage  SampleTime=-1
  电池温度(℃) : ToWorkspace  VariableName=Bat_temp_oC  SampleTime=-1
  电池组剩余容量 : ToWorkspace  VariableName=Bat_cap_Ah  SampleTime=-1
  电池组衰退容量 : ToWorkspace  VariableName=Bat_cap_degradation_Ah  SampleTime=-1
  电池衰退严重因子 : ToWorkspace  VariableName=Bat_age_severity_factor  SampleTime=-1
  计算实际寿命 : Subsystem
  计算电池寿命(标准条件下) : Subsystem
  wires:
  SOC/1 -> Switch1/2, Scope7/1, ×/1, Switch2/2, 计算实际寿命/3(SOC)
  Alpha2/1 -> Switch1/1
  Alpha1/1 -> Switch1/3
  Beta2/1 -> Switch2/1
  Beta1/1 -> Switch2/3
  Switch1/1 -> ×/2
  Switch2/1 -> Alpha*SOC+Beta/2
  ×/1 -> Alpha*SOC+Beta/1
  Rg/1 -> R*T/1
  ℃->开氏温度(绝对温度)/1 -> R*T/2
  Ic=I/Q0/1 -> Scope1/1, Ic/2, 计算实际寿命/2(倍率), 充放电倍率/1
  Alpha*SOC+Beta/1 -> R*T2/1, Scope3/1
  Constant/1 -> -31700+152.5*Ic/1
  Ic/1 -> -31700+152.5*Ic/2
  Constant1/1 -> Ic/1
  -31700+152.5*Ic/1 -> x1/1
  R*T/1 -> x1/2
  Math Function2/1 -> R*T2/2, Scope3/2
  x1/1 -> Math Function2/1
  Math Function1/1 -> R*T2/3, Scope3/3
  R*T2/1 -> Scope/1, Display1/1, 电池容量衰退百分比 (累计值：%)/1, %/1
  Abs/1 -> Ic=I/Q0/2, Ah/1, Scope2/1
  Integrator/1 -> Math Function1/1, 安时通量/1
  Temp (oC)/1 -> 计算实际寿命/1(温度), 电池温度(℃)/1, ℃->开氏温度(绝对温度)/1
  Constant2/1 -> ℃->开氏温度(绝对温度)/2
  %/1 -> Qloss_cell,Ah/1
  温度/1 -> 计算电池寿命(标准条件下)/1(标准温度)
  标准倍率/1 -> 计算电池寿命(标准条件下)/2(标准倍率)
  标准SOC/1 -> 计算电池寿命(标准条件下)/3(标准SOC)
  Product/1 -> 电池衰退严重因子/1, Scope10/1
  计算实际寿命/1(Bat_life_nom) -> 实际寿命&标称寿命/1, Product/1
  计算电池寿命(标准条件下)/1(Bat_life_act) -> Product/2, 实际寿命&标称寿命/2
  I(A)/1 -> Abs/1
  Cell nominal capacity (Ah)/1 -> Qloss_cell,Ah/2, Ic=I/Q0/1
  Qcell->Qbat/1 -> Q0-Qloss/1, 电池组衰退容量/1
  Qloss_cell,Ah/1 -> Qcell->Qbat/1
  Battery capacity (Ah)/1 -> Q0-Qloss/2
  Q0-Qloss/1 -> 电池组剩余容量/1
  Ah/1 -> Integrator/1
  Constant3/1 -> Math Function1/2

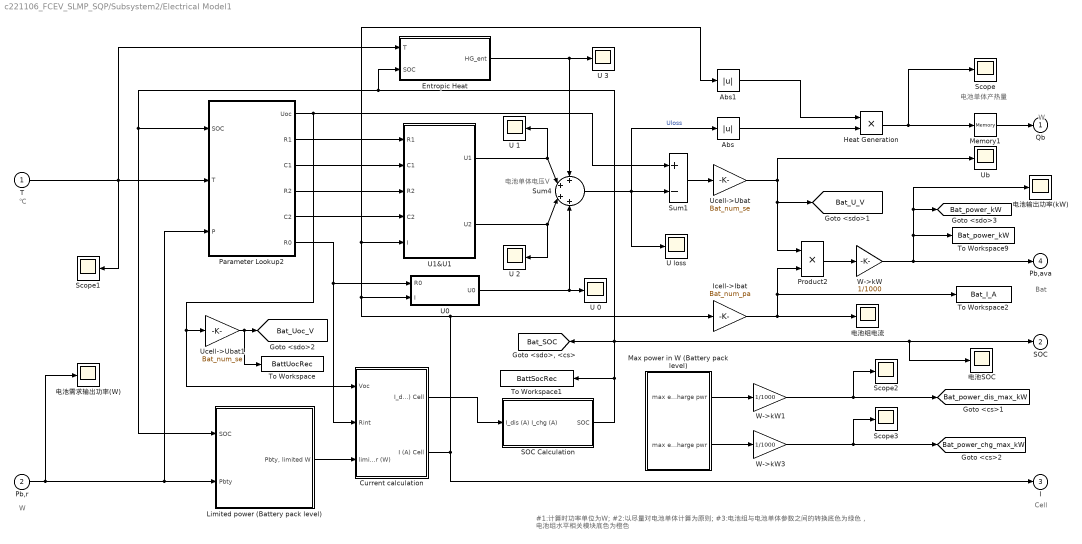
== system c221106_FCEV_SLMP_SQP/Subsystem2/Electrical Model1 ==
  note: Bat
  note: Cell
  note: W
  note: ℃
  note: #1:计算时功率单位为W;
      | #2:以尽量对电池单体计算为原则;
      | #3:电池组与电池单体参数之间的转换底色为绿色， 电池组水平相关模块底色为橙色
  note: W
  note: 电池单体产热量
  note: 电池单体电压V
  T : Inport
  Pb,r : Inport  Port=2
  Abs : Abs  SaturateOnIntegerOverflow=off
  Abs1 : Abs  SaturateOnIntegerOverflow=off
  Current calculation : Subsystem
  Entropic Heat : Subsystem
  Heat Generation : Product  RndMeth=Zero
  Icell->Ibat : Gain  Gain=Bat_num_pa  SaturateOnIntegerOverflow=on  OutDataTypeStr=Inherit: Same as input  ParamDataTypeStr=Inherit: Same as input
  Limited power (Battery pack level) : Subsystem
  Max power in W (Battery pack level) : Subsystem
  Memory1 : Memory  InheritSampleTime=on
  Parameter Lookup2 : Subsystem
  Product2 : Product  RndMeth=Zero
  SOC Calculation : Subsystem
  Scope{,1..3} (4 alike) : Scope
  Sum1 : Sum  Inputs=+-
  Sum4 : Sum  Inputs=++++
  To Workspace : ToWorkspace  VariableName=BattUocRec  SaveFormat=Timeseries  SampleTime=-1
  To Workspace1 : ToWorkspace  VariableName=BattSocRec  SampleTime=-1
  To Workspace2 : ToWorkspace  VariableName=Bat_I_A  SampleTime=-1
  To Workspace9 : ToWorkspace  VariableName=Bat_power_kW  SampleTime=-1
  U {0..3} (4 alike) : Scope
  U loss : Scope
  U0 : Subsystem
  U1&U1 : Subsystem
  Ub : Scope
  Ucell->Ubat : Gain  Gain=Bat_num_se  SaturateOnIntegerOverflow=on  OutDataTypeStr=Inherit: Same as input  ParamDataTypeStr=Inherit: Same as input
  Ucell->Ubat1 : Gain  Gain=Bat_num_se  SaturateOnIntegerOverflow=on  OutDataTypeStr=Inherit: Same as input  ParamDataTypeStr=Inherit: Same as input
  W->kW : Gain  Gain=1/1000  SaturateOnIntegerOverflow=on  OutDataTypeStr=Inherit: Same as input  ParamDataTypeStr=Inherit: Same as input
  W->kW1 : Gain  Gain=1/1000  SaturateOnIntegerOverflow=on  OutDataTypeStr=Inherit: Same as input  ParamDataTypeStr=Inherit: Same as input
  W->kW3 : Gain  Gain=1/1000  SaturateOnIntegerOverflow=on  OutDataTypeStr=Inherit: Same as input  ParamDataTypeStr=Inherit: Same as input
  电池SOC : Scope
  电池组电流 : Scope
  电池输出功率(kW) : Scope
  电池需求输出功率(W) : Scope
  Qb : Outport  InitialOutput=0
  SOC : Outport  Port=2  InitialOutput=0
  I : Outport  Port=3  InitialOutput=0
  Pb,ava : Outport  Port=4  InitialOutput=0
  tag scope: Bat_SOC=global, Bat_U_V=global, Bat_Uoc_V=global, Bat_power_chg_max_kW=global, Bat_power_dis_max_kW=global, Bat_power_kW=global
  wires:
  Parameter Lookup2/2(R1) -> U1&U1/1(R1)
  Parameter Lookup2/3(C1) -> U1&U1/2(C1)
  Parameter Lookup2/4(R2) -> U1&U1/3(R2)
  Parameter Lookup2/5(C2) -> U1&U1/4(C2)
  Parameter Lookup2/6(R0) -> U0/1(R0), Current calculation/2(Rint)
  U1&U1/1(U1) -> Sum4/2, U 1/1
  U1&U1/2(U2) -> U 2/1, Sum4/3
  Ucell->Ubat/1 -> Product2/1, [Bat_U_V], Ub/1
  Entropic Heat/1(HG_ent) -> U 3/1, Sum4/1
  Product2/1 -> W->kW/1
  W->kW/1 -> 电池输出功率(kW)/1, [Bat_power_kW], To Workspace9/1, Pb,ava/1
  Memory1/1 -> Qb/1
  Heat Generation/1 -> Scope/1, Memory1/1
  Current calculation/1(I_dis (A) I_chg (A) Cell) -> SOC Calculation/1(I_dis (A) I_chg (A))
  T/1 -> Scope1/1, Entropic Heat/1(T), Parameter Lookup2/2(T)
  Pb,r/1 -> 电池需求输出功率(W)/1, Limited power (Battery pack level)/2(Pbty), Parameter Lookup2/3(P)
  Icell->Ibat/1 -> Product2/2, To Workspace2/1, 电池组电流/1
  W->kW1/1 -> Scope2/1, [Bat_power_dis_max_kW]
  W->kW3/1 -> Scope3/1, [Bat_power_chg_max_kW]
  Max power in W (Battery pack level)/1(max ess discharge pwr) -> W->kW1/1
  Max power in W (Battery pack level)/2(max ess charge pwr) -> W->kW3/1
  Parameter Lookup2/1(Uoc) -> Sum1/1, Ucell->Ubat1/1, Current calculation/1(Voc)
  Ucell->Ubat1/1 -> To Workspace/1, [Bat_Uoc_V]
  Limited power (Battery pack level)/1("Pbty, limited W") -> Current calculation/3(limited output power (W))
  SOC Calculation/1(SOC) -> 电池SOC/1, SOC/1, [Bat_SOC], Entropic Heat/2(SOC), Limited power (Battery pack level)/1(SOC), Parameter Lookup2/1(SOC), To Workspace1/1
  Current calculation/2(I (A) Cell) -> Abs1/1, U1&U1/5(I), U0/2(I), Icell->Ibat/1, I/1
  U0/1(U0) -> U 0/1, Sum4/4
  Sum4/1 -> U loss/1, Abs/1, Sum1/2  "Uloss"
  Sum1/1 -> Ucell->Ubat/1
  Abs/1 -> Heat Generation/2
  Abs1/1 -> Heat Generation/1

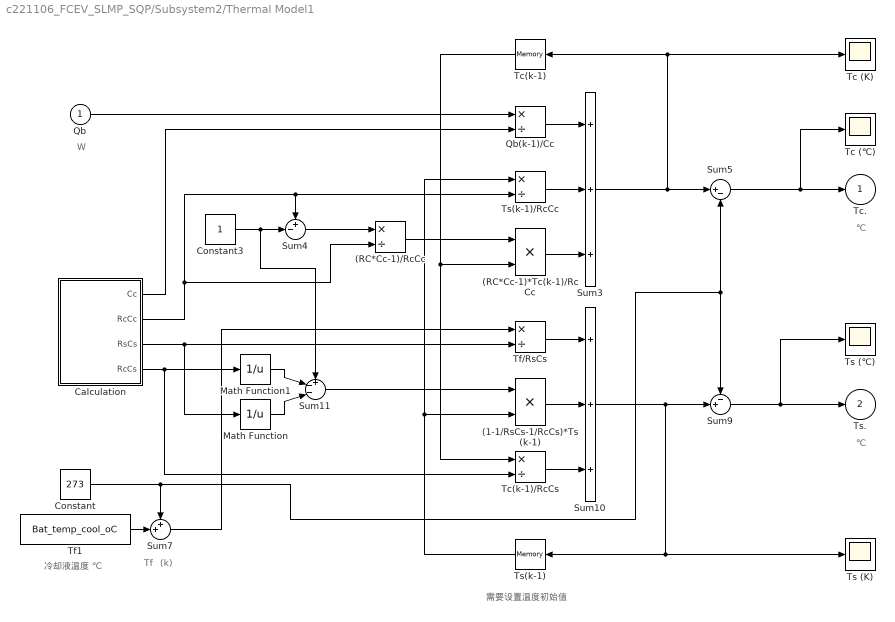
== system c221106_FCEV_SLMP_SQP/Subsystem2/Thermal Model1 ==
  note: 需要设置温度初始值
  note: W
  note: Tf
  note: (k)
  note: 冷却液温度 ℃
  note: ℃
  note: ℃
  Qb : Inport
  (1-1/RsCs-1/RcCs)*Ts(k-1) : Product  Inputs=**  RndMeth=Zero
  (RC*Cc-1)*Tc(k-1)/RcCc : Product  Inputs=**  RndMeth=Zero
  (RC*Cc-1)/RcCc : Product  Inputs=*/  RndMeth=Zero
  Calculation : Subsystem
  Constant : Constant  Value=273
  Constant3 : Constant
  Math Function : Math  Operator=reciprocal  SignedPower=on
  Math Function1 : Math  Operator=reciprocal  SignedPower=on
  Qb(k-1)/Cc : Product  Inputs=*/  RndMeth=Zero
  Sum10 : Sum  Inputs=+++
  Sum11 : Sum  Inputs=+--|
  Sum3 : Sum  Inputs=+++
  Sum4 : Sum  Inputs=+-|
  Sum5 : Sum  Inputs=|+-
  Sum7 : Sum  Inputs=++|
  Sum9 : Sum  Inputs=-+|
  Tc (K) : Scope
  Tc (℃) : Scope
  Tc(k-1) : Memory  InitialCondition=Bat_temp_amb_oC+273.15  InheritSampleTime=on
  Tc(k-1)/RcCs : Product  Inputs=*/  RndMeth=Zero
  Tf/RsCs : Product  Inputs=*/  RndMeth=Zero
  Tf1 : Constant  Value=Bat_temp_cool_oC
  Ts (K) : Scope
  Ts (℃) : Scope
  Ts(k-1) : Memory  InitialCondition=Bat_temp_amb_oC+273.15  InheritSampleTime=on
  Ts(k-1)/RcCc : Product  Inputs=*/  RndMeth=Zero
  Tc. : Outport
  Ts. : Outport  Port=2
  wires:
  Calculation/1(Cc) -> Qb(k-1)/Cc/2
  Calculation/2(RcCc) -> (RC*Cc-1)/RcCc/2, Ts(k-1)/RcCc/2, Sum4/1
  Constant3/1 -> Sum11/1, Sum4/2
  Sum4/1 -> (RC*Cc-1)/RcCc/1
  Qb(k-1)/Cc/1 -> Sum3/1
  Ts(k-1)/RcCc/1 -> Sum3/2
  Tf1/1 -> Sum7/2
  Calculation/3(RsCs) -> Tf/RsCs/2, Math Function/1
  Sum7/1 -> Tf/RsCs/1
  Tf/RsCs/1 -> Sum10/1
  Calculation/4(RcCs) -> Tc(k-1)/RcCs/2, Math Function1/1
  Math Function1/1 -> Sum11/2
  Math Function/1 -> Sum11/3
  (1-1/RsCs-1/RcCs)*Ts(k-1)/1 -> Sum10/2
  Sum11/1 -> (1-1/RsCs-1/RcCs)*Ts(k-1)/1
  Tc(k-1)/RcCs/1 -> Sum10/3
  Sum3/1 -> Sum5/1, Tc(k-1)/1, Tc (K)/1
  Constant/1 -> Sum9/1, Sum5/2, Sum7/1
  Sum5/1 -> Tc (℃)/1, Tc./1
  Sum10/1 -> Sum9/2, Ts(k-1)/1, Ts (K)/1
  Sum9/1 -> Ts./1, Ts (℃)/1
  Ts(k-1)/1 -> Ts(k-1)/RcCc/1, (1-1/RsCs-1/RcCs)*Ts(k-1)/2
  (RC*Cc-1)*Tc(k-1)/RcCc/1 -> Sum3/3
  (RC*Cc-1)/RcCc/1 -> (RC*Cc-1)*Tc(k-1)/RcCc/1
  Tc(k-1)/1 -> Tc(k-1)/RcCs/1, (RC*Cc-1)*Tc(k-1)/RcCc/2
  Qb/1 -> Qb(k-1)/Cc/1

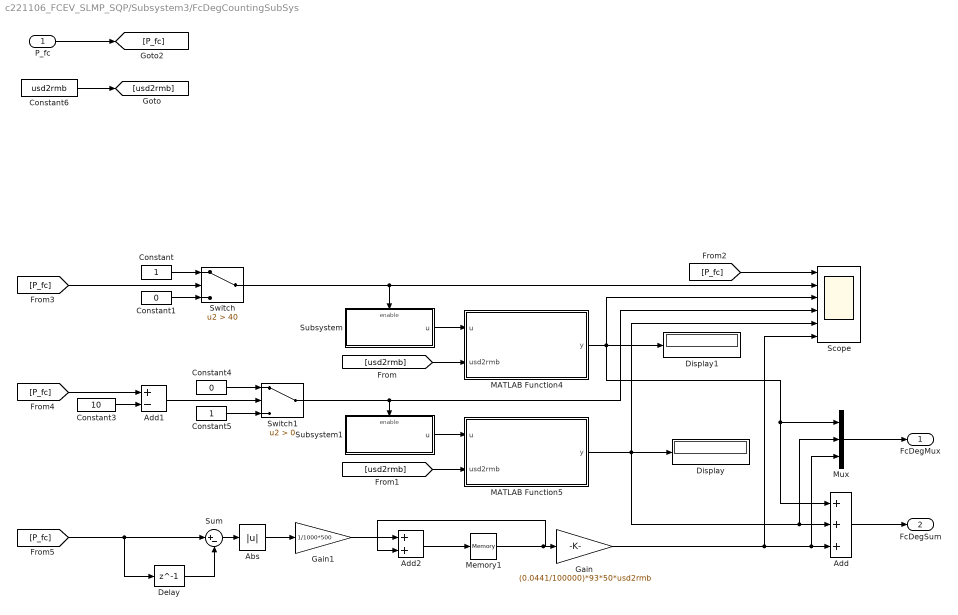
== system c221106_FCEV_SLMP_SQP/Subsystem3/FcDegCountingSubSys ==
  P_fc : Inport
  Abs : Abs  SaturateOnIntegerOverflow=off
  Add : Sum  Inputs=+++
  Add1 : Sum  Inputs=+-
  Add2 : Sum
  Constant : Constant
  Constant1 : Constant  Value=0
  Constant3 : Constant  Value=10
  Constant4 : Constant  Value=0
  Constant5 : Constant
  Constant6 : Constant  Value=usd2rmb
  Delay : Delay  DelayLength=1
  Display : Display
  Display1 : Display
  Gain : Gain  Gain=(0.0441/100000)*93*50*usd2rmb
  Gain1 : Gain  Gain=1/1000*500
  MATLAB Function4 : MATLAB Function  TreatAsAtomicUnit=on
  MATLAB Function5 : MATLAB Function  TreatAsAtomicUnit=on
  Memory1 : Memory
  Mux : Mux  Inputs=3
  Scope : Scope  NumInputPorts=6
  Subsystem : Subsystem
  Subsystem1 : Subsystem
  Sum : Sum  Inputs=|+-
  Switch : Switch  Criteria=u2 > Threshold  Threshold=40  SaturateOnIntegerOverflow=off  InputSameDT=off
  Switch1 : Switch  Criteria=u2 > Threshold  SaturateOnIntegerOverflow=off  InputSameDT=off
  FcDegMux : Outport
  FcDegSum : Outport  Port=2
  wires:
  MATLAB Function5/1(y) -> Scope/5, Display/1, Mux/2, Add/2
  Constant3/1 -> Add1/2
  Constant5/1 -> Switch1/3
  Switch1/1 -> Scope/4, Subsystem1/Enable
  Add1/1 -> Switch1/2
  Subsystem/1(u) -> MATLAB Function4/1(u)
  Constant/1 -> Switch/1
  [usd2rmb] -> MATLAB Function4/2(usd2rmb)
  Constant1/1 -> Switch/3
  Constant4/1 -> Switch1/1
  [usd2rmb] -> MATLAB Function5/2(usd2rmb)
  Switch/1 -> Scope/2, Subsystem/Enable
  P_fc/1 -> [P_fc]
  Subsystem1/1(u) -> MATLAB Function5/1(u)
  MATLAB Function4/1(y) -> Scope/3, Mux/1, Add/1, Display1/1
  Constant6/1 -> [usd2rmb]
  [P_fc] -> Scope/1
  Gain/1 -> Scope/6, Mux/3, Add/3
  Gain1/1 -> Add2/1
  Add2/1 -> Memory1/1
  Sum/1 -> Abs/1
  Abs/1 -> Gain1/1
  Delay/1 -> Sum/2
  Memory1/1 -> Gain/1, Add2/2
  [P_fc] -> Delay/1, Sum/1
  [P_fc] -> Switch/2
  [P_fc] -> Add1/1
  Add/1 -> FcDegSum/1
  Mux/1 -> FcDegMux/1

== system c221106_FCEV_SLMP_SQP/Subsystem3/Fuel Rate Calculation1 ==
  note: Transient load response
  fc pwr : Inport
  "FC hydrogen consumption rate " : Lookup_n-D  NumberOfTableDimensions=1  BreakpointsForDimension1=FC_ori_power_kW  Table=FC_ori_fuel_rate_gps  RndMeth=Simplest
  fcv_H2_rate (g/s)1 : Outport
  wires:
  fc pwr/1 -> "FC hydrogen consumption rate "/1
  "FC hydrogen consumption rate "/1 -> fcv_H2_rate (g/s)1/1  "fcv_hot_H2_hist"

== system c221106_FCEV_SLMP_SQP/Subsystem3/Fuel cell efficiency calculation ==
  note: Carryover
  note: Transient load response
  fc power : Inport
  "FC efficiency " : Lookup_n-D  NumberOfTableDimensions=1  BreakpointsForDimension1=FC_ori_power_kW  Table=FC_ori_eff  RndMeth=Simplest
  "fc_eff " : Outport
  wires:
  "FC efficiency "/1 -> "fc_eff "/1
  fc power/1 -> "FC efficiency "/1

== system c221106_FCEV_SLMP_SQP/Subsystem3/Power Calculation ==
  note: Transient load response
  fc on : Inport
  Power command (kW) : Inport  Port=2
  "   " : Constant  Value=0
  Switch2 : Switch  Threshold=0.5
  Power output (kW) : Outport
  wires:
  "   "/1 -> Switch2/3
  Power command (kW)/1 -> Switch2/1
  fc on/1 -> Switch2/2
  Switch2/1 -> Power output (kW)/1

== system c221106_FCEV_SLMP_SQP/Subsystem4/VehModel_Pred+1 ==
  note: CarryOver
  Pred_v1 : Inport
  Enable : EnablePort
  Gain : Gain  Gain=3.6
  Power bus : Subsystem
  主减及变速器模型 : Subsystem
  整车动力学模型 : Subsystem
  车轮模型 : Subsystem
  驱动电机模型 : Subsystem
  PredPwr_1 : Outport
  wires:
  主减及变速器模型/1(drive torque (Nm) speed (rad/s) brike torque (Nm) req'd at input side of final drive) -> 驱动电机模型/1(drive torque (Nm) speed (rad/s) brake torque (Nm) req'd at motor)
  驱动电机模型/1(drive power (kW) brake power (kW) req'd motor input power (电功率)) -> Power bus/1(drive power (kW) brake power (kW) req at power bus)
  整车动力学模型/1(需求驱动力N 目标车速m/s 需求制动力N) -> 车轮模型/1("tractive force, brake force and speed req'd of tire/road interface 需求驱动力N 目标车速m/s 需求制动力N")
  车轮模型/1(drive torque (Nm) speed (rad/s) brake torque (Nm) req'd from drivetrain into axle) -> 主减及变速器模型/1(drive torque (Nm) speed (rad/s) brake torque (Nm) req'd at output side of final drive)
  Pred_v1/1 -> Gain/1
  Power bus/1(drive power (kW)/brake power (kW) req from power sources) -> PredPwr_1/1
  Gain/1 -> 整车动力学模型/1(需求车速 km/h)

== system c221106_FCEV_SLMP_SQP/Subsystem4/VehModel_Pred+2 ==
  note: CarryOver
  Pred_v2 : Inport
  Pred_v1 : Inport  Port=2
  Enable : EnablePort
  Gain : Gain  Gain=3.6
  Gain1 : Gain  Gain=3.6
  Power bus : Subsystem
  主减及变速器模型 : Subsystem
  整车动力学模型 : Subsystem
  车轮模型 : Subsystem
  驱动电机模型 : Subsystem
  PredPwr_2 : Outport
  wires:
  主减及变速器模型/1(drive torque (Nm) speed (rad/s) brike torque (Nm) req'd at input side of final drive) -> 驱动电机模型/1(drive torque (Nm) speed (rad/s) brake torque (Nm) req'd at motor)
  驱动电机模型/1(drive power (kW) brake power (kW) req'd motor input power (电功率)) -> Power bus/1(drive power (kW) brake power (kW) req at power bus)
  整车动力学模型/1(需求驱动力N 目标车速m/s 需求制动力N) -> 车轮模型/1("tractive force, brake force and speed req'd of tire/road interface 需求驱动力N 目标车速m/s 需求制动力N")
  车轮模型/1(drive torque (Nm) speed (rad/s) brake torque (Nm) req'd from drivetrain into axle) -> 主减及变速器模型/1(drive torque (Nm) speed (rad/s) brake torque (Nm) req'd at output side of final drive)
  Pred_v2/1 -> Gain/1
  Power bus/1(drive power (kW)/brake power (kW) req from power sources) -> PredPwr_2/1
  Gain/1 -> 整车动力学模型/1(需求车速 km/h)
  Pred_v1/1 -> Gain1/1
  Gain1/1 -> 整车动力学模型/2(Temp)

== system c221106_FCEV_SLMP_SQP/Subsystem4/VehModel_Pred+3 ==
  note: CarryOver
  Pred_v3 : Inport
  Pred_v2 : Inport  Port=2
  Enable : EnablePort
  Gain : Gain  Gain=3.6
  Gain1 : Gain  Gain=3.6
  Power bus : Subsystem
  主减及变速器模型 : Subsystem
  整车动力学模型 : Subsystem
  车轮模型 : Subsystem
  驱动电机模型 : Subsystem
  PredPwr_3 : Outport
  wires:
  主减及变速器模型/1(drive torque (Nm) speed (rad/s) brike torque (Nm) req'd at input side of final drive) -> 驱动电机模型/1(drive torque (Nm) speed (rad/s) brake torque (Nm) req'd at motor)
  驱动电机模型/1(drive power (kW) brake power (kW) req'd motor input power (电功率)) -> Power bus/1(drive power (kW) brake power (kW) req at power bus)
  整车动力学模型/1(需求驱动力N 目标车速m/s 需求制动力N) -> 车轮模型/1("tractive force, brake force and speed req'd of tire/road interface 需求驱动力N 目标车速m/s 需求制动力N")
  车轮模型/1(drive torque (Nm) speed (rad/s) brake torque (Nm) req'd from drivetrain into axle) -> 主减及变速器模型/1(drive torque (Nm) speed (rad/s) brake torque (Nm) req'd at output side of final drive)
  Pred_v3/1 -> Gain/1
  Power bus/1(drive power (kW)/brake power (kW) req from power sources) -> PredPwr_3/1
  Gain/1 -> 整车动力学模型/1(需求车速 km/h)
  Pred_v2/1 -> Gain1/1
  Gain1/1 -> 整车动力学模型/2(需求车速 km/h1)
